simulink model "BLOCK"  (Simulink 7.9)
settings: Solver=ode45  StartTime=0.0  StopTime=6  RelTol=1e-3
settings Model: Creator=Nick  LastModifiedBy=Nick

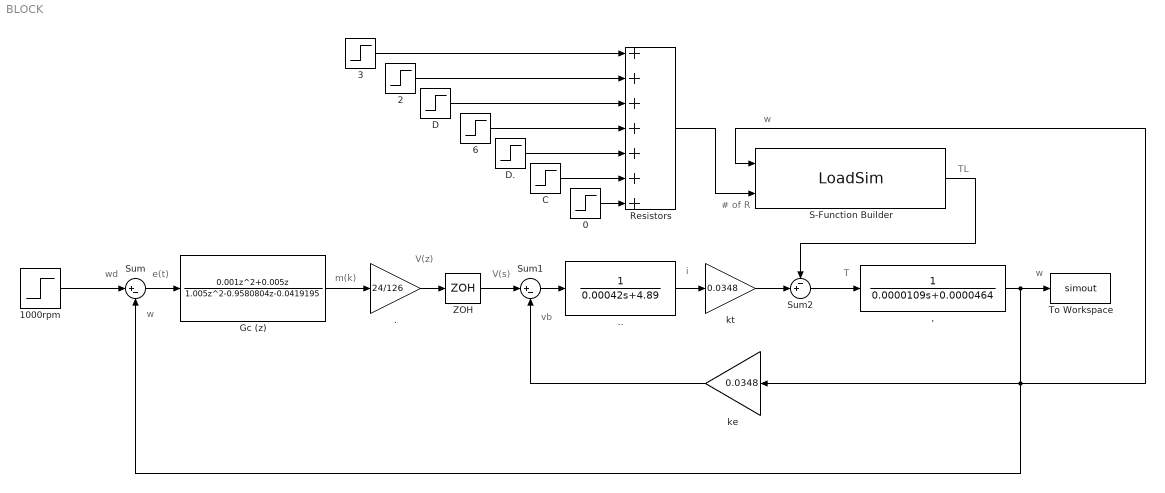
== system BLOCK ==
  note: wd
  note: e(t)
  note: m(k)
  note: V(z)
  note: V(s)
  note: vb
  note: w
  note: i
  note: T
  note: w
  note: w
  note: # of R
  note: TL
  , : TransferFcn  Denominator=[0.0000109 0.0000464]
  . : Gain  Gain=24/126  SampleTime=0.004
  .. : TransferFcn  Denominator=[0.00042 4.89]
  0 : Step  Time=5.6  After=-12  SampleTime=0.004
  1000rpm : Step  Time=0  After=1000  SampleTime=0.004
  2 : Step  Time=1.6  After=-1  SampleTime=0.004
  3 : Step  Time=0.8  After=3  SampleTime=0.004
  6 : Step  Time=3.2  After=-7  SampleTime=0.004
  C : Step  Time=4.8  After=-1  SampleTime=0.004
  D : Step  Time=2.4  After=11  SampleTime=0.004
  D. : Step  Time=4.0  After=7  SampleTime=0.004
  Gc (z) : DiscreteTransferFcn  Tag=z  Numerator=[0.001 0.005 0]  Denominator=[1.005 -0.9580804 -0.0419195]  SampleTime=0.004
  Resistors : Sum  Inputs=+++++++
  S-Function Builder : S-Function  InitFcn=try, set_param(gcb,'FunctionName','LoadSim'), end,  FunctionName=LoadSim  SFunctionModules=LoadSim_wrapper  WizardData=DataTag0  EnableBusSupport=off  mask(S-Function Builder){}
      mask init:
      | val = [[.9  0.75 0.75 1 1 .9 .9 1]',[1 1 0.75 0.75 .9 .9 1 .9]'];try , sys = get_param(gcb,'SfunBuilderFcnName');if isempty(sys), sys = get_param(gcb,'FunctionName'); end,catch, sys = get_param(gcb,'FunctionName'); end
      settings: CopyFcn=set_param(gcbh,'LinkStatus','none')  PreSaveFcn=try, set_param(gcb,'FunctionName','LoadSim'), end  OpenFcn=sfunctionwizard(gcbh)
      mask Display: plot(val(:,1),val(:,2)),disp(sys), port_label('input',1,'u0'), port_label('input',2,'u1'), port_label('output',1,'y0')
  Sum : Sum  Inputs=|+-  SampleTime=0.004
  Sum1 : Sum  Inputs=|+-  SampleTime=0.004
  Sum2 : Sum  Inputs=-+|
  To Workspace : ToWorkspace  VariableName=simout  SampleTime=0.004
  ZOH : ZeroOrderHold  SampleTime=0.004
  ke : Gain  Gain=0.0348  SampleTime=0.004
  kt : Gain  Gain=0.0348  SampleTime=0.004
  wires:
  Sum/1 -> Gc (z)/1
  Gc (z)/1 -> ./1
  ./1 -> ZOH/1
  ZOH/1 -> Sum1/1
  ke/1 -> Sum1/2
  Sum1/1 -> ../1
  ../1 -> kt/1
  ,/1 -> Sum/2, ke/1, S-Function Builder/1, To Workspace/1
  kt/1 -> Sum2/2
  Sum2/1 -> ,/1
  1000rpm/1 -> Sum/1
  S-Function Builder/1 -> Sum2/1
  Resistors/1 -> S-Function Builder/2
  C/1 -> Resistors/6
  D./1 -> Resistors/5
  6/1 -> Resistors/4
  D/1 -> Resistors/3
  2/1 -> Resistors/2
  3/1 -> Resistors/1
  0/1 -> Resistors/7
